simulink model "AWGN_SNR_test"  (R2014b)
settings: Solver=ode45  StartTime=0.0  StopTime=1e-2  RelTol=1e-3
libraries: dspstat3 x2, commdigbbndam3 x2, commchan3 x1, commrandsrc2 x1
settings Model: Creator=Tim-UML  LastModifiedBy=Tim-UML

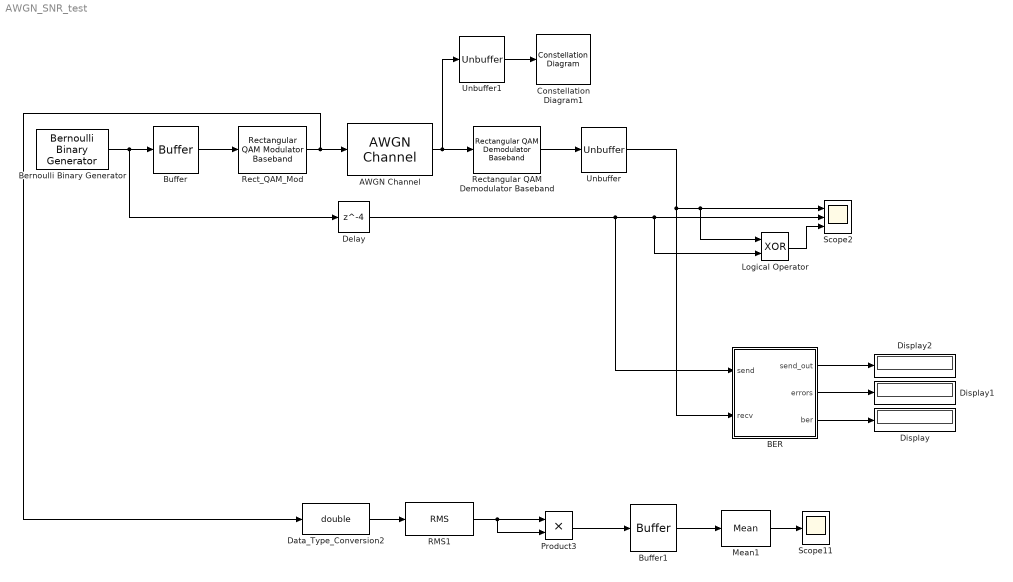
== system AWGN_SNR_test ==
  AWGN Channel : commchan3/AWGN Channel  InputProcessing=Columns as channels (frame based)  seed=1604198  noiseMode="Signal to noise ratio  (SNR)"  EbNodB=18  EsNodB=10  SNRdB=18  bitsPerSym=56  Ps=10  Tsym=1120e-9  variance=1
  BER : Subsystem
  Bernoulli Binary Generator : commrandsrc2/Bernoulli Binary Generator  P=0.5  seed=1604198  Ts=20e-9  frameBased=off  sampPerFrame=1  orient=off  outDataType=boolean
      settings: AttributesFormatString=|
      | Sample Time= %<Ts>
      | Prob zero=%<P>
  Buffer : Buffer  N=4  TreatMby1Signals=One channel
  Buffer1 : Buffer  N=128  TreatMby1Signals=One channel
  Constellation Diagram1 : ConstellationDiagram
  Data_Type_Conversion2 : DataTypeConversion  OutDataTypeStr=double  RndMeth=Convergent
  Delay : Delay  DelayLength=4  InitialCondition=0
  Display : Display
      settings: Format=short_e
  Display1 : Display
      settings: Format=short_e
  Display2 : Display
      settings: Format=short_e
  Logical Operator : Logic  Operator=XOR  AllPortsSameDT=off  OutDataTypeStr=boolean
  Mean1 : dspstat3/Mean  run=off  reset_popup=None  InputProcessing=Columns as channels (frame based)  directionMode=Entire input  dimension=1  treatSBRowAsCol=on  roiEnable=off  roiType=Rectangles  roiPortion=Entire ROI  roiOutput=Individual statistics for each ROI  roiFlag=off  outputDataTypeStr=Inherit: Same as accumulator  outputLastDataTypeStr=Inherit: Same as accumulator  outputMin=[]  outputMax=[]  roundingMode=Floor  overflowMode=off
  Product3 : Product
  RMS1 : dspstat3/RMS  run=off  reset_popup=None  InputProcessing=Columns as channels (frame based)  directionMode=Each column  dimension=1  treatSBRowAsCol=on
  Rect_QAM_Mod : commdigbbndam3/Rectangular QAM Modulator Baseband  M=16  InType=Bit  Enc=Gray  Mapping=[0:15]  PowType=Min. distance between symbols  MinDist=2  AvgPow=1  PeakPow=1  Ph=0  outDtype=double  outWordLen=16  outUDDataType=sfix(12)  outFracLenMode=User-defined  outFracLen=6
  Rectangular QAM Demodulator Baseband : commdigbbndam3/Rectangular QAM Demodulator Baseband  M=16  PowType=Min. distance between symbols  MinDist=2  AvgPow=1  PeakPow=1  Ph=0  Dec=Gray  Mapping=[0:15]  OutType=Bit  DecType=Hard decision  VarSource=Dialog  Variance=1  outDtype1=boolean  outDtype2=Inherit via internal rule  derotateFactorWordLen=16  denormFactorWordLen=16  prodOutWordLen=32  prodOutRoundingMode=Convergent  prodOutOverflowMode=Saturate  sumWordLen=32
  Scope11 : Scope
      settings: TimeRange=2e-05  YMin=72.5  YMax=76.5  SaveName=ScopeData119
  Scope2 : Scope  NumInputPorts=3
      settings: TimeRange=2e-05  YMin=-10~-8~-5  YMax=8~8~5  SaveName=ScopeData53
  Unbuffer : Unbuffer  SampleBasedProcessing=Same as frame based
  Unbuffer1 : Unbuffer  SampleBasedProcessing=Same as frame based
  wires:
  Buffer/1 -> Rect_QAM_Mod/1
  Rect_QAM_Mod/1 -> Data_Type_Conversion2/1, AWGN Channel/1
  AWGN Channel/1 -> Unbuffer1/1, Rectangular QAM Demodulator Baseband/1
  Rectangular QAM Demodulator Baseband/1 -> Unbuffer/1
  Bernoulli Binary Generator/1 -> Delay/1, Buffer/1
  Logical Operator/1 -> Scope2/3
  Delay/1 -> BER/1(send), Logical Operator/2, Scope2/2
  BER/1(send_out) -> Display2/1
  BER/2(errors) -> Display1/1
  BER/3(ber) -> Display/1
  Unbuffer/1 -> BER/2(recv), Logical Operator/1, Scope2/1
  Unbuffer1/1 -> Constellation Diagram1/1
  Data_Type_Conversion2/1 -> RMS1/1
  RMS1/1 -> Product3/2, Product3/1
  Mean1/1 -> Scope11/1
  Buffer1/1 -> Mean1/1
  Product3/1 -> Buffer1/1

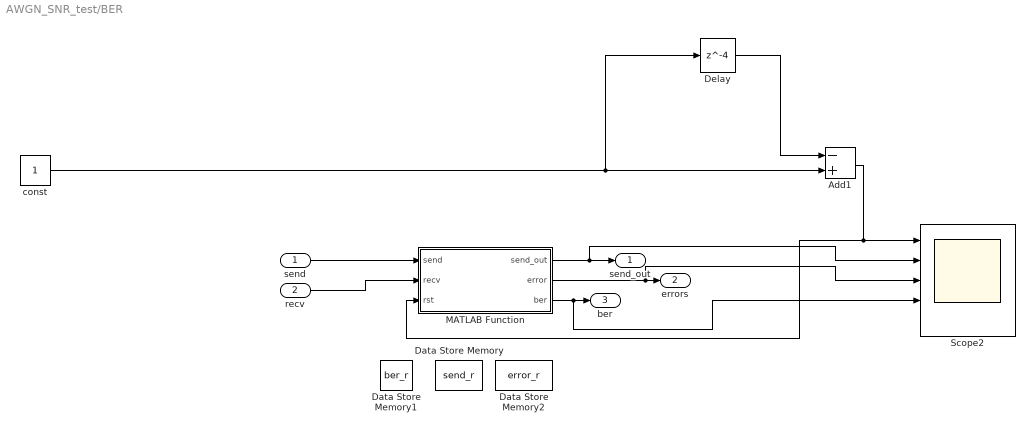
== system AWGN_SNR_test/BER ==
  send : Inport
  recv : Inport  Port=2
  Add1 : Sum  Inputs=-+
  Data Store Memory : DataStoreMemory  DataStoreName=send_r  OutDataTypeStr=double
  Data Store Memory1 : DataStoreMemory  DataStoreName=ber_r  OutDataTypeStr=double
  Data Store Memory2 : DataStoreMemory  DataStoreName=error_r  OutDataTypeStr=double
  Delay : Delay  DelayLength=4  InitialCondition=0
  MATLAB Function : MATLAB Function  TreatAsAtomicUnit=on  SystemSampleTime=20e-9
  Scope2 : Scope  NumInputPorts=5
      settings: TimeRange=3e-05  YMin=0~0~0~0~0  YMax=1~1~1~1~1  SaveName=ScopeData115
  const : Constant  SampleTime=20e-9
  send_out : Outport
  errors : Outport  Port=2
  ber : Outport  Port=3
  wires:
  MATLAB Function/2(error) -> Scope2/3, errors/1
  MATLAB Function/1(send_out) -> Scope2/2, send_out/1
  recv/1 -> MATLAB Function/2(recv)
  MATLAB Function/3(ber) -> Scope2/4, ber/1
  send/1 -> MATLAB Function/1(send)
  const/1 -> Delay/1, Add1/2
  Add1/1 -> MATLAB Function/3(rst), Scope2/1
  Delay/1 -> Add1/1

== matlab function AWGN_SNR_test/BER/MATLAB Function ==
  data: send input; send_out output; error output; recv input; ber_r data_store_memory; send_r data_store_memory; error_r data_store_memory; ber output; rst input
function [send_out,error,ber] = ber_ratio (  send, recv, rst)

global ber_r;
global send_r;
global error_r;

send_r=send_r+1;

if send ~= recv
    error_r = error_r+1;
    ber_r = error_r/send_r;
end


if rst == 1
    ber_r=0;
    send_r=0;
    error_r=0;
end

send_out = send_r;
error = error_r;
ber = ber_r;
end
